simulink model "Irrigation_Control_System"  (R2023a)
settings: Solver=VariableStepAuto  StartTime=0.0  StopTime=inf  RelTol=1e-3
settings Model: Creator=Mass  LastModifiedBy=Mass

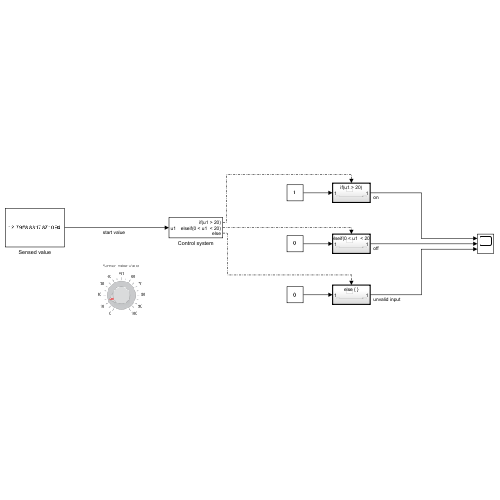
[thumbnail: Simulink's stored preview of the top-level diagram]
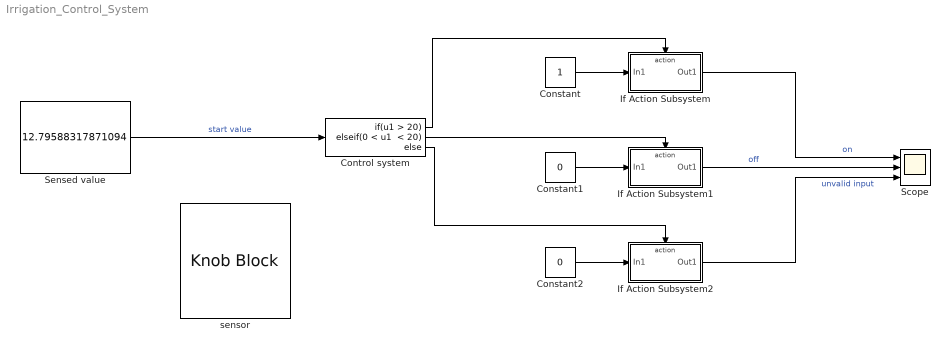
== system Irrigation_Control_System ==
  Constant : Constant
  Constant1 : Constant  Value=0
  Constant2 : Constant  Value=0
  Control system : If  IfExpression=u1 > 20  ElseIfExpressions="0 < u1  < 20"
  If Action Subsystem : Subsystem  TreatAsAtomicUnit=on
  If Action Subsystem1 : Subsystem  TreatAsAtomicUnit=on
  If Action Subsystem2 : Subsystem  TreatAsAtomicUnit=on
  Scope : Scope  NumInputPorts=3
  Sensed value : Constant  Value=12.79588317871094
  sensor : KnobBlock
  wires:
  Sensed value/1 -> Control system/1  "start value"
  Control system/1 -> If Action Subsystem/Action
  Control system/2 -> If Action Subsystem1/Action
  Control system/3 -> If Action Subsystem2/Action
  Constant/1 -> If Action Subsystem/1(In1)
  Constant1/1 -> If Action Subsystem1/1(In1)
  Constant2/1 -> If Action Subsystem2/1(In1)
  If Action Subsystem/1(Out1) -> Scope/1  "on"
  If Action Subsystem1/1(Out1) -> Scope/2  "off"
  If Action Subsystem2/1(Out1) -> Scope/3  "unvalid input"

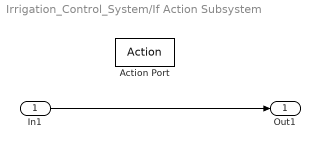
== system Irrigation_Control_System/If Action Subsystem ==
  In1 : Inport
  Action Port : ActionPort  ActionPortLabel=if(u1 > 20)
  Out1 : Outport
  wires:
  In1/1 -> Out1/1

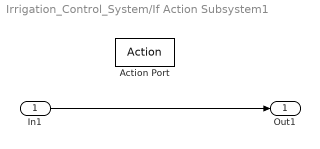
== system Irrigation_Control_System/If Action Subsystem1 ==
  In1 : Inport
  Action Port : ActionPort  ActionPortLabel="elseif(0 < u1  < 20)"
  Out1 : Outport
  wires:
  In1/1 -> Out1/1

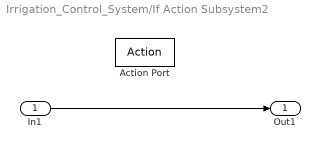
== system Irrigation_Control_System/If Action Subsystem2 ==
  In1 : Inport
  Action Port : ActionPort  ActionPortLabel=else
  Out1 : Outport
  wires:
  In1/1 -> Out1/1
